simulink model "m5_das_ext"  (R2015b)
settings: Solver=FixedStepAuto  SolverMode=SingleTasking  StartTime=0.0  StopTime=10.0  RelTol=1e-3
undefined symbols (not defined in the file): DiscIntNeverNeededParam
libraries: simulink x5
settings Model: Creator=Capstone  LastModifiedBy=muscari.s

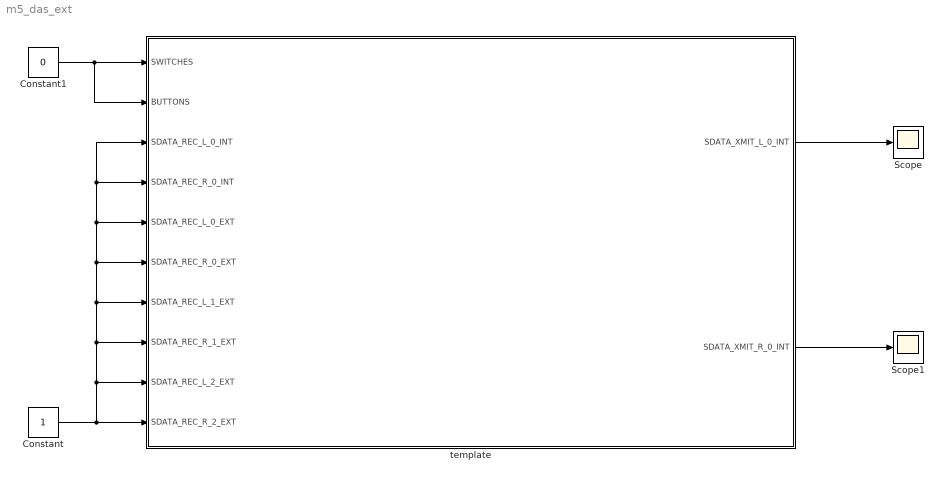
== system m5_das_ext ==
  Constant : Constant  OutDataTypeStr=int32  SampleTime=-1  LockScale=on
  Constant1 : Constant  Value=0  OutDataTypeStr=uint32  SampleTime=-1  LockScale=on
  Scope : Scope
  Scope1 : Scope
  template : Subsystem  TreatAsAtomicUnit=on
  wires:
  template/2(SDATA_XMIT_R_0_INT) -> Scope1/1
  template/1(SDATA_XMIT_L_0_INT) -> Scope/1
  Constant1/1 -> template/1(SWITCHES), template/2(BUTTONS)
  Constant/1 -> template/10(SDATA_REC_R_2_EXT), template/9(SDATA_REC_L_2_EXT), template/8(SDATA_REC_R_1_EXT), template/7(SDATA_REC_L_1_EXT), template/6(SDATA_REC_R_0_EXT), template/5(SDATA_REC_L_0_EXT), template/4(SDATA_REC_R_0_INT), template/3(SDATA_REC_L_0_INT)

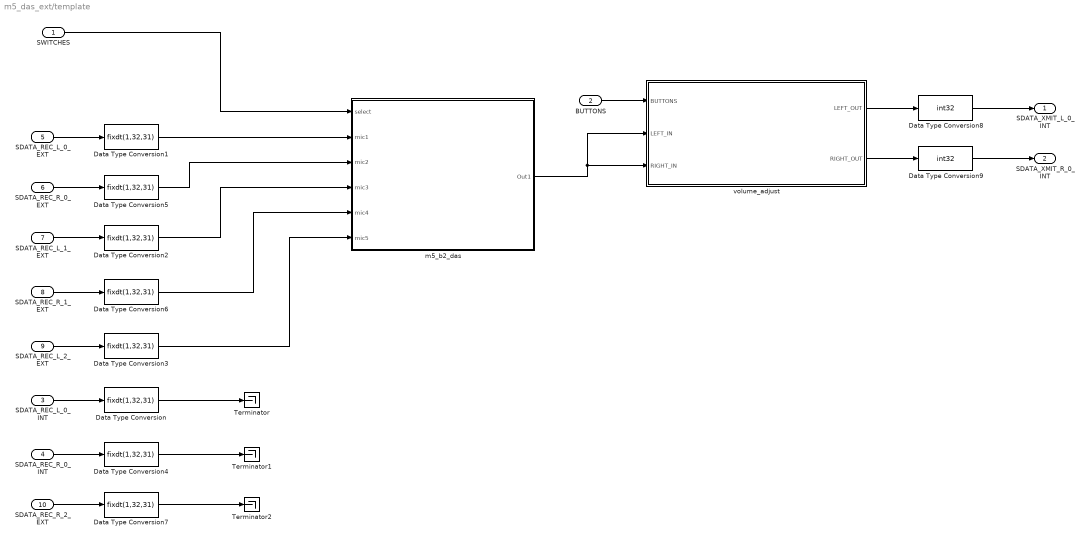
== system m5_das_ext/template ==
  SWITCHES : Inport
  BUTTONS : Inport  Port=2
  SDATA_REC_L_0_INT : Inport  Port=3
  SDATA_REC_R_0_INT : Inport  Port=4
  SDATA_REC_L_0_EXT : Inport  Port=5
  SDATA_REC_R_0_EXT : Inport  Port=6
  SDATA_REC_L_1_EXT : Inport  Port=7
  SDATA_REC_R_1_EXT : Inport  Port=8
  SDATA_REC_L_2_EXT : Inport  Port=9
  SDATA_REC_R_2_EXT : Inport  Port=10
  Data Type Conversion{,1..7} (8 alike) : DataTypeConversion  OutDataTypeStr=fixdt(1,32,31)  ConvertRealWorld=Stored Integer (SI)  RndMeth=Zero
  Data Type Conversion8 : DataTypeConversion  OutDataTypeStr=int32  ConvertRealWorld=Stored Integer (SI)  SaturateOnIntegerOverflow=on  RndMeth=Zero
  Data Type Conversion9 : DataTypeConversion  OutDataTypeStr=int32  ConvertRealWorld=Stored Integer (SI)  SaturateOnIntegerOverflow=on  RndMeth=Zero
  Terminator : Terminator
  Terminator1 : Terminator
  Terminator2 : Terminator
  m5_b2_das : Subsystem
  volume_adjust : Subsystem
  SDATA_XMIT_L_0_INT : Outport
  SDATA_XMIT_R_0_INT : Outport  Port=2
  wires:
  SDATA_REC_L_0_INT/1 -> Data Type Conversion/1
  SDATA_REC_R_0_INT/1 -> Data Type Conversion4/1
  SDATA_REC_L_0_EXT/1 -> Data Type Conversion1/1
  SDATA_REC_R_0_EXT/1 -> Data Type Conversion5/1
  SDATA_REC_L_1_EXT/1 -> Data Type Conversion2/1
  SDATA_REC_R_1_EXT/1 -> Data Type Conversion6/1
  SDATA_REC_L_2_EXT/1 -> Data Type Conversion3/1
  SDATA_REC_R_2_EXT/1 -> Data Type Conversion7/1
  BUTTONS/1 -> volume_adjust/1(BUTTONS)
  volume_adjust/1(LEFT_OUT) -> Data Type Conversion8/1
  volume_adjust/2(RIGHT_OUT) -> Data Type Conversion9/1
  Data Type Conversion8/1 -> SDATA_XMIT_L_0_INT/1
  Data Type Conversion9/1 -> SDATA_XMIT_R_0_INT/1
  SWITCHES/1 -> m5_b2_das/1(select)
  m5_b2_das/1(Out1) -> volume_adjust/2(LEFT_IN), volume_adjust/3(RIGHT_IN)
  Data Type Conversion7/1 -> Terminator2/1
  Data Type Conversion1/1 -> m5_b2_das/2(mic1)
  Data Type Conversion5/1 -> m5_b2_das/3(mic2)
  Data Type Conversion2/1 -> m5_b2_das/4(mic3)
  Data Type Conversion6/1 -> m5_b2_das/5(mic4)
  Data Type Conversion3/1 -> m5_b2_das/6(mic5)
  Data Type Conversion/1 -> Terminator/1
  Data Type Conversion4/1 -> Terminator1/1

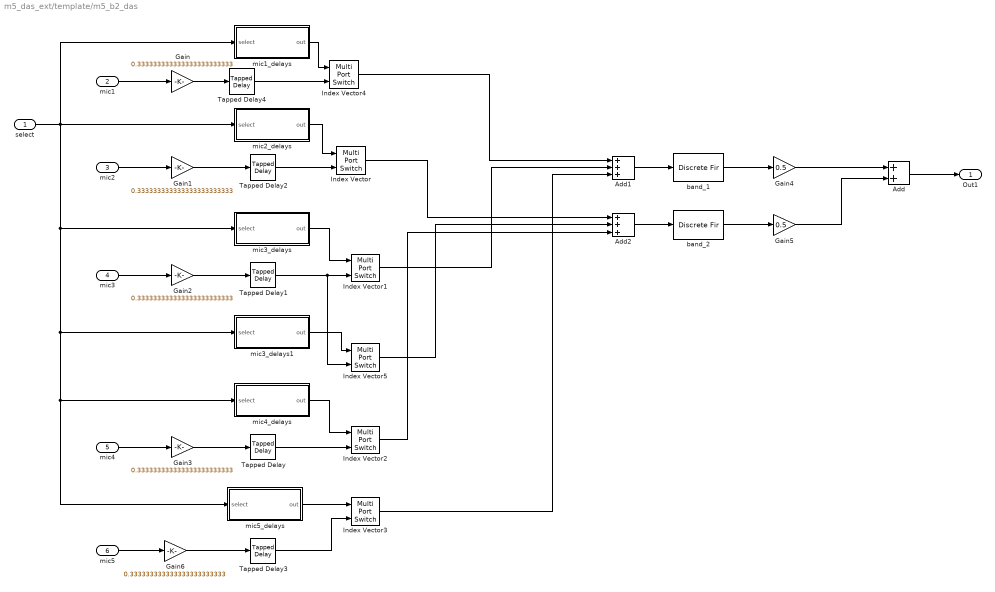
== system m5_das_ext/template/m5_b2_das ==
  select : Inport
  mic1 : Inport  Port=2
  mic2 : Inport  Port=3
  mic3 : Inport  Port=4
  mic4 : Inport  Port=5
  mic5 : Inport  Port=6
  Add : Sum  OutDataTypeStr=Inherit: Inherit via back propagation  RndMeth=Zero
  Add1 : Sum  Inputs=+++  OutDataTypeStr=Inherit: Inherit via back propagation  RndMeth=Zero
  Add2 : Sum  Inputs=+++  OutDataTypeStr=Inherit: Inherit via back propagation  RndMeth=Zero
  Gain{,1..3,6} (5 alike) : Gain  Gain=0.333333333333333333333333  ParamDataTypeStr=fixdt(1,32,31)  OutDataTypeStr=Inherit: Inherit via back propagation  RndMeth=Zero
  Gain4 : Gain  Gain=0.5  ParamDataTypeStr=fixdt(1,32,31)  OutDataTypeStr=Inherit: Inherit via back propagation  RndMeth=Zero
  Gain5 : Gain  Gain=0.5  ParamDataTypeStr=fixdt(1,32,31)  OutDataTypeStr=Inherit: Inherit via back propagation  RndMeth=Zero
  Index Vector{,1..5} (6 alike) : MultiPortSwitch  DataPortOrder=Zero-based contiguous  Inputs=1  zeroidx=on  OutDataTypeStr=Inherit: Inherit via back propagation  RndMeth=Zero
  Tapped Delay : simulink/Discrete/Tapped Delay  vinit=0.0  samptime=-1  NumDelays=17  DelayOrder=Newest  includeCurrent=on
  Tapped Delay1 : simulink/Discrete/Tapped Delay  vinit=0.0  samptime=-1  NumDelays=23  DelayOrder=Newest  includeCurrent=on
  Tapped Delay2 : simulink/Discrete/Tapped Delay  vinit=0.0  samptime=-1  NumDelays=17  DelayOrder=Newest  includeCurrent=on
  Tapped Delay3 : simulink/Discrete/Tapped Delay  vinit=0.0  samptime=-1  NumDelays=47  DelayOrder=Newest  includeCurrent=on
  Tapped Delay4 : simulink/Discrete/Tapped Delay  vinit=0.0  samptime=-1  NumDelays=47  DelayOrder=Newest  includeCurrent=on
  band_1 : DiscreteFir  FilterStructure=Direct form symmetric  Coefficients=[-0.0006782323736677226 -0.00061797501410385913 -0.00055397321805590496 -0.00048323247815375899 -0.0004028708790337593 -0.00031134760707579243 -0.00020971779606389519 -0.00010278232418469137 5.3436904881575911e-19 8.3960710390948516e-05 0.00012913286531009868 0.0001106975285270993 0 -0.00023387312629336585 -0.00062201085466718272 -0.0011931884772806989 -0.0019711128359718205 -0.0029715765047669592 -0.004199718624744401 -0.005647601071181548 -0.0072923056704523453 -0.0090947407353308349 -0.010999313649242089 -0.012934581980254817 -0.014814940943676075 -0.016543343055917401 -0.018014980247362096 -0.019121793633739462 -0.019757615819354583 -0.019823699110911527 -0.019234344027896737 -0.017922319003094409 -0.015843756286986907 -0.012982221866819705 -0.0093516886044415284 -0.004998190536744853 3.2646934950337606e-18 0.0055337554288432044 0.011466036402723352 0.017636310418650814 0.023866277092597258 0.029966655648355277 0.035744726086331557 0.041012267278278738 0.045593505981502414 0.049332682487998818 0.052100852097979732 0.053801576321740811 0.054375211888126766 0.053801576321740811 0.052100852097979732 0.049332682487998818 0.045593505981502414 0.041012267278278738 0.035744726086331557 0.029966655648355277 0.023866277092597258 0.017636310418650814 0.011466036402723352 0.0055337554288432044 3.2646934950337606e-18 -0.004998190536744853 -0.0093516886044415284 -0.012982221866819705 -0.015843756286986907 -0.017922319003094409 -0.019234344027896737 -0.019823699110911527 -0.019757615819354583 -0.019121793633739462 -0.018014980247362096 -0.016543343055917401 -0.014814940943676075 -0.012934581980254817 -0.010999313649242089 -0.0090947407353308349 -0.0072923056704523453 -0.005647601071181548 -0.004199718624744401 -0.0029715765047669592 -0.0019711128359718205 -0.0011931884772806989 -0.00062201085466718272 -0.00023387312629336585 0 0.0001106975285270993 0.00012913286531009868 8.3960710390948516e-05 5.3436904881575911e-19 -0.00010278232418469137 -0.00020971779606389519 -0.00031134760707579243 -0.0004028708790337593 -0.00048323247815375899 -0.00055397321805590496 -0.00061797501410385913 -0.0006782323736677226]  TapSumDataTypeStr=fixdt(true,33,31)  CoefDataTypeStr=fixdt(true,32,31)  ProductDataTypeStr=fixdt(true,32,31)  AccumDataTypeStr=fixdt(true,32,31)  OutDataTypeStr=fixdt(true,32,31)  RndMeth=Zero
  band_2 : DiscreteFir  FilterStructure=Direct form symmetric  Coefficients=[0.00031148187044047459 -5.1095487798674356e-05 -0.00038181538543607328 -0.00062770468081234799 -0.00074248208966874556 -0.00070004998252385145 -0.00051178880868063385 -0.00024029641821307493 1.3497652502458736e-18 6.2855354767847132e-05 -0.00018821474507956884 -0.00082507757949582753 -0.0018036973576697544 -0.0029373522174964005 -0.0039121114215135214 -0.0043514130535061441 -0.0039203448488945537 -0.0024435921126518823 3.3068411990632952e-18 0.0030435832447575401 0.0060838439066612541 0.008418897314846626 0.0094448958102664009 0.0088589350919107673 0.0068038414189030769 0.0038972922777800981 0.0011143345940897462 -0.00046666289418714551 6.8520344440706088e-18 0.0027988407275439764 0.0074343909211899992 0.01260813889409973 0.016432926965007474 0.016863521806897715 0.01225654659999127 0.0019235994936369317 -0.013475782186410821 -0.031831181698260456 -0.049836435118945893 -0.063583988307230208 -0.0693890532919961 -0.064664003280160934 -0.048634089538675054 -0.022707689666544836 0.0096145175855820303 0.043302394792267433 0.072729178597249478 0.09277940187005515 0.099888435657650002 0.09277940187005515 0.072729178597249478 0.043302394792267433 0.0096145175855820303 -0.022707689666544836 -0.048634089538675054 -0.064664003280160934 -0.0693890532919961 -0.063583988307230208 -0.049836435118945893 -0.031831181698260456 -0.013475782186410821 0.0019235994936369317 0.01225654659999127 0.016863521806897715 0.016432926965007474 0.01260813889409973 0.0074343909211899992 0.0027988407275439764 6.8520344440706088e-18 -0.00046666289418714551 0.0011143345940897462 0.0038972922777800981 0.0068038414189030769 0.0088589350919107673 0.0094448958102664009 0.008418897314846626 0.0060838439066612541 0.0030435832447575401 3.3068411990632952e-18 -0.0024435921126518823 -0.0039203448488945537 -0.0043514130535061441 -0.0039121114215135214 -0.0029373522174964005 -0.0018036973576697544 -0.00082507757949582753 -0.00018821474507956884 6.2855354767847132e-05 1.3497652502458736e-18 -0.00024029641821307493 -0.00051178880868063385 -0.00070004998252385145 -0.00074248208966874556 -0.00062770468081234799 -0.00038181538543607328 -5.1095487798674356e-05 0.00031148187044047459]  TapSumDataTypeStr=fixdt(true,33,31)  CoefDataTypeStr=fixdt(true,32,31)  ProductDataTypeStr=fixdt(true,32,31)  AccumDataTypeStr=fixdt(true,32,31)  OutDataTypeStr=fixdt(true,32,31)  RndMeth=Zero
  mic1_delays : Subsystem
  mic2_delays : Subsystem
  mic3_delays : Subsystem
  mic3_delays1 : Subsystem
  mic4_delays : Subsystem
  mic5_delays : Subsystem
  Out1 : Outport
  wires:
  mic1/1 -> Gain/1
  mic2/1 -> Gain1/1
  mic3/1 -> Gain2/1
  mic4/1 -> Gain3/1
  Gain1/1 -> Tapped Delay2/1
  Gain2/1 -> Tapped Delay1/1
  Gain3/1 -> Tapped Delay/1
  Tapped Delay2/1 -> Index Vector/2
  select/1 -> mic2_delays/1(select), mic1_delays/1(select), mic3_delays/1(select), mic3_delays1/1(select), mic4_delays/1(select), mic5_delays/1(select)
  Tapped Delay1/1 -> Index Vector5/2, Index Vector1/2
  Tapped Delay/1 -> Index Vector2/2
  band_1/1 -> Gain4/1
  band_2/1 -> Gain5/1
  Gain4/1 -> Add/1
  Gain5/1 -> Add/2
  mic5/1 -> Gain6/1
  Tapped Delay3/1 -> Index Vector3/2
  Add/1 -> Out1/1
  Gain6/1 -> Tapped Delay3/1
  Add1/1 -> band_1/1
  Add2/1 -> band_2/1
  Tapped Delay4/1 -> Index Vector4/2
  Gain/1 -> Tapped Delay4/1
  mic1_delays/1(out) -> Index Vector4/1
  Index Vector4/1 -> Add1/1
  mic3_delays/1(out) -> Index Vector1/1
  Index Vector1/1 -> Add1/2
  mic5_delays/1(out) -> Index Vector3/1
  Index Vector3/1 -> Add1/3
  mic2_delays/1(out) -> Index Vector/1
  mic4_delays/1(out) -> Index Vector2/1
  mic3_delays1/1(out) -> Index Vector5/1
  Index Vector5/1 -> Add2/2
  Index Vector/1 -> Add2/1
  Index Vector2/1 -> Add2/3

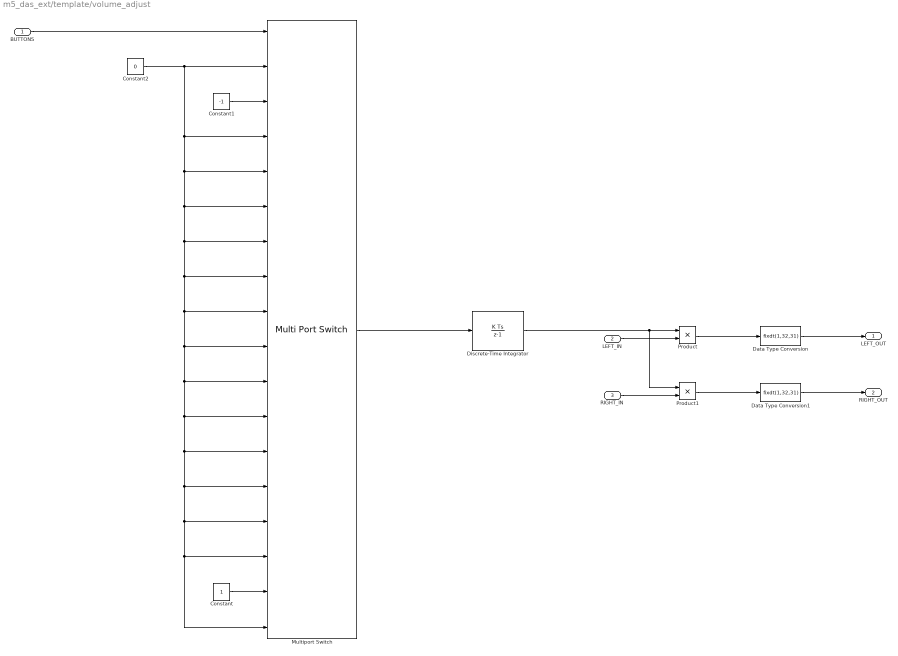
== system m5_das_ext/template/volume_adjust ==
  BUTTONS : Inport
  LEFT_IN : Inport  Port=2
  RIGHT_IN : Inport  Port=3
  Constant : Constant  OutDataTypeStr=fixdt(1,64,31)  SampleTime=-1
  Constant1 : Constant  Value=-1  OutDataTypeStr=fixdt(1,64,31)  SampleTime=-1
  Constant2 : Constant  Value=0  OutDataTypeStr=fixdt(1,64,31)  SampleTime=-1
  Data Type Conversion : DataTypeConversion  OutDataTypeStr=fixdt(1,32,31)  RndMeth=Zero
  Data Type Conversion1 : DataTypeConversion  OutDataTypeStr=fixdt(1,32,31)  RndMeth=Zero
  Discrete-Time Integrator : DiscreteIntegrator  gainval=0.00005  InitialCondition=1  OutDataTypeStr=fixdt(1,64,31)  RndMeth=Zero  SaturateOnIntegerOverflow=on  LimitOutput=on  UpperSaturationLimit=10000  LowerSaturationLimit=0  ICPrevOutput=DiscIntNeverNeededParam  ICPrevScaledInput=DiscIntNeverNeededParam
  Multiport Switch : MultiPortSwitch  Inputs=16  DataPortIndices={16,2}  DataPortForDefault=Additional data port  DiagnosticForDefault=None  OutDataTypeStr=Inherit: Inherit via back propagation  RndMeth=Zero
  Product : Product  OutDataTypeStr=Inherit: Inherit via back propagation  RndMeth=Zero
  Product1 : Product  OutDataTypeStr=Inherit: Inherit via back propagation  RndMeth=Zero
  LEFT_OUT : Outport
  RIGHT_OUT : Outport  Port=2
  wires:
  Multiport Switch/1 -> Discrete-Time Integrator/1
  BUTTONS/1 -> Multiport Switch/1
  Discrete-Time Integrator/1 -> Product1/1, Product/1
  LEFT_IN/1 -> Product/2
  RIGHT_IN/1 -> Product1/2
  Product/1 -> Data Type Conversion/1
  Product1/1 -> Data Type Conversion1/1
  Data Type Conversion/1 -> LEFT_OUT/1
  Data Type Conversion1/1 -> RIGHT_OUT/1
  Constant/1 -> Multiport Switch/17
  Constant1/1 -> Multiport Switch/3
  Constant2/1 -> Multiport Switch/2, Multiport Switch/18, Multiport Switch/16, Multiport Switch/15, Multiport Switch/14, Multiport Switch/13, Multiport Switch/12, Multiport Switch/11, Multiport Switch/10, Multiport Switch/9, Multiport Switch/8, Multiport Switch/7, Multiport Switch/6, Multiport Switch/5, Multiport Switch/4

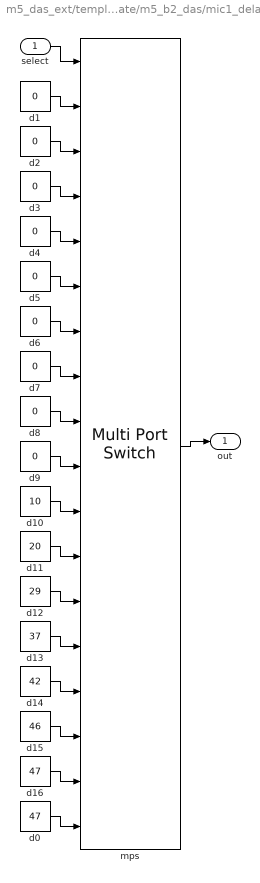
== system m5_das_ext/template/m5_b2_das/mic1_delays ==
  select : Inport
  d0 : Constant  Value=47  OutDataTypeStr=uint16  SampleTime=-1
  d{1..9} (9 alike) : Constant  Value=0  OutDataTypeStr=uint16  SampleTime=-1
  d10 : Constant  Value=10  OutDataTypeStr=uint16  SampleTime=-1
  d11 : Constant  Value=20  OutDataTypeStr=uint16  SampleTime=-1
  d12 : Constant  Value=29  OutDataTypeStr=uint16  SampleTime=-1
  d13 : Constant  Value=37  OutDataTypeStr=uint16  SampleTime=-1
  d14 : Constant  Value=42  OutDataTypeStr=uint16  SampleTime=-1
  d15 : Constant  Value=46  OutDataTypeStr=uint16  SampleTime=-1
  d16 : Constant  Value=47  OutDataTypeStr=uint16  SampleTime=-1
  mps : MultiPortSwitch  DataPortOrder=Zero-based contiguous  Inputs=16  DataPortForDefault=Additional data port  DiagnosticForDefault=None  OutDataTypeStr=Inherit: Inherit via back propagation  RndMeth=Zero  InputSameDT=on
  out : Outport
  wires:
  select/1 -> mps/1
  mps/1 -> out/1
  d1/1 -> mps/2
  d2/1 -> mps/3
  d3/1 -> mps/4
  d4/1 -> mps/5
  d5/1 -> mps/6
  d6/1 -> mps/7
  d7/1 -> mps/8
  d8/1 -> mps/9
  d9/1 -> mps/10
  d10/1 -> mps/11
  d11/1 -> mps/12
  d12/1 -> mps/13
  d13/1 -> mps/14
  d14/1 -> mps/15
  d15/1 -> mps/16
  d16/1 -> mps/17
  d0/1 -> mps/18

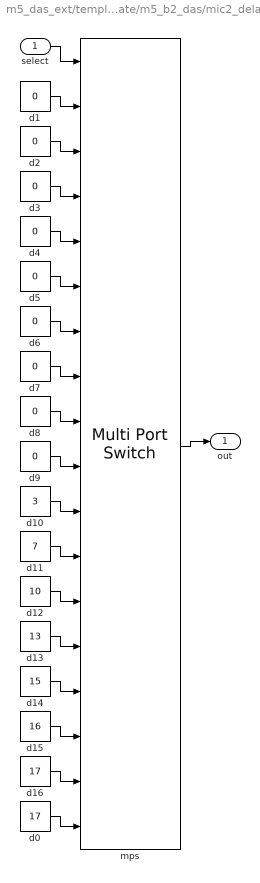
== system m5_das_ext/template/m5_b2_das/mic2_delays ==
  select : Inport
  d0 : Constant  Value=17  OutDataTypeStr=uint16  SampleTime=-1
  d{1..9} (9 alike) : Constant  Value=0  OutDataTypeStr=uint16  SampleTime=-1
  d10 : Constant  Value=3  OutDataTypeStr=uint16  SampleTime=-1
  d11 : Constant  Value=7  OutDataTypeStr=uint16  SampleTime=-1
  d12 : Constant  Value=10  OutDataTypeStr=uint16  SampleTime=-1
  d13 : Constant  Value=13  OutDataTypeStr=uint16  SampleTime=-1
  d14 : Constant  Value=15  OutDataTypeStr=uint16  SampleTime=-1
  d15 : Constant  Value=16  OutDataTypeStr=uint16  SampleTime=-1
  d16 : Constant  Value=17  OutDataTypeStr=uint16  SampleTime=-1
  mps : MultiPortSwitch  DataPortOrder=Zero-based contiguous  Inputs=16  DataPortForDefault=Additional data port  DiagnosticForDefault=None  OutDataTypeStr=Inherit: Inherit via back propagation  RndMeth=Zero  InputSameDT=on
  out : Outport
  wires:
  select/1 -> mps/1
  mps/1 -> out/1
  d1/1 -> mps/2
  d2/1 -> mps/3
  d3/1 -> mps/4
  d4/1 -> mps/5
  d5/1 -> mps/6
  d6/1 -> mps/7
  d7/1 -> mps/8
  d8/1 -> mps/9
  d9/1 -> mps/10
  d10/1 -> mps/11
  d11/1 -> mps/12
  d12/1 -> mps/13
  d13/1 -> mps/14
  d14/1 -> mps/15
  d15/1 -> mps/16
  d16/1 -> mps/17
  d0/1 -> mps/18

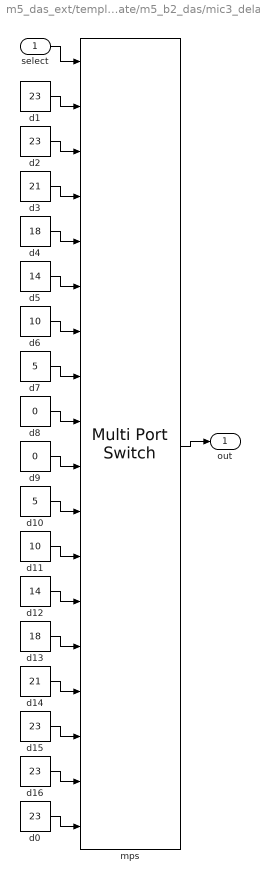
== system m5_das_ext/template/m5_b2_das/mic3_delays ==
  select : Inport
  d{0..2,15..16} (5 alike) : Constant  Value=23  OutDataTypeStr=uint16  SampleTime=-1
  d10 : Constant  Value=5  OutDataTypeStr=uint16  SampleTime=-1
  d11 : Constant  Value=10  OutDataTypeStr=uint16  SampleTime=-1
  d12 : Constant  Value=14  OutDataTypeStr=uint16  SampleTime=-1
  d13 : Constant  Value=18  OutDataTypeStr=uint16  SampleTime=-1
  d14 : Constant  Value=21  OutDataTypeStr=uint16  SampleTime=-1
  d3 : Constant  Value=21  OutDataTypeStr=uint16  SampleTime=-1
  d4 : Constant  Value=18  OutDataTypeStr=uint16  SampleTime=-1
  d5 : Constant  Value=14  OutDataTypeStr=uint16  SampleTime=-1
  d6 : Constant  Value=10  OutDataTypeStr=uint16  SampleTime=-1
  d7 : Constant  Value=5  OutDataTypeStr=uint16  SampleTime=-1
  d8 : Constant  Value=0  OutDataTypeStr=uint16  SampleTime=-1
  d9 : Constant  Value=0  OutDataTypeStr=uint16  SampleTime=-1
  mps : MultiPortSwitch  DataPortOrder=Zero-based contiguous  Inputs=16  DataPortForDefault=Additional data port  DiagnosticForDefault=None  OutDataTypeStr=Inherit: Inherit via back propagation  RndMeth=Zero  InputSameDT=on
  out : Outport
  wires:
  select/1 -> mps/1
  mps/1 -> out/1
  d1/1 -> mps/2
  d2/1 -> mps/3
  d3/1 -> mps/4
  d4/1 -> mps/5
  d5/1 -> mps/6
  d6/1 -> mps/7
  d7/1 -> mps/8
  d8/1 -> mps/9
  d9/1 -> mps/10
  d10/1 -> mps/11
  d11/1 -> mps/12
  d12/1 -> mps/13
  d13/1 -> mps/14
  d14/1 -> mps/15
  d15/1 -> mps/16
  d16/1 -> mps/17
  d0/1 -> mps/18

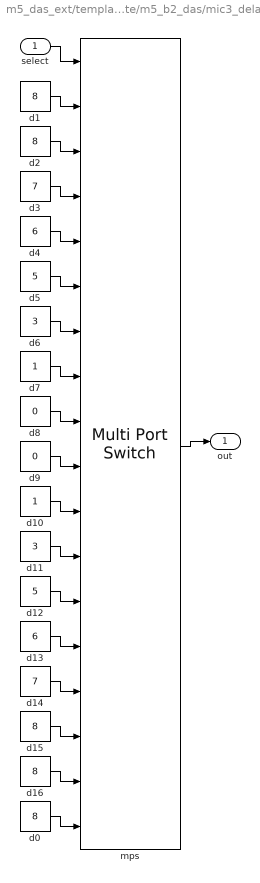
== system m5_das_ext/template/m5_b2_das/mic3_delays1 ==
  select : Inport
  d{0..2,15..16} (5 alike) : Constant  Value=8  OutDataTypeStr=uint16  SampleTime=-1
  d10 : Constant  OutDataTypeStr=uint16  SampleTime=-1
  d11 : Constant  Value=3  OutDataTypeStr=uint16  SampleTime=-1
  d12 : Constant  Value=5  OutDataTypeStr=uint16  SampleTime=-1
  d13 : Constant  Value=6  OutDataTypeStr=uint16  SampleTime=-1
  d14 : Constant  Value=7  OutDataTypeStr=uint16  SampleTime=-1
  d3 : Constant  Value=7  OutDataTypeStr=uint16  SampleTime=-1
  d4 : Constant  Value=6  OutDataTypeStr=uint16  SampleTime=-1
  d5 : Constant  Value=5  OutDataTypeStr=uint16  SampleTime=-1
  d6 : Constant  Value=3  OutDataTypeStr=uint16  SampleTime=-1
  d7 : Constant  OutDataTypeStr=uint16  SampleTime=-1
  d8 : Constant  Value=0  OutDataTypeStr=uint16  SampleTime=-1
  d9 : Constant  Value=0  OutDataTypeStr=uint16  SampleTime=-1
  mps : MultiPortSwitch  DataPortOrder=Zero-based contiguous  Inputs=16  DataPortForDefault=Additional data port  DiagnosticForDefault=None  OutDataTypeStr=Inherit: Inherit via back propagation  RndMeth=Zero  InputSameDT=on
  out : Outport
  wires:
  select/1 -> mps/1
  mps/1 -> out/1
  d1/1 -> mps/2
  d2/1 -> mps/3
  d3/1 -> mps/4
  d4/1 -> mps/5
  d5/1 -> mps/6
  d6/1 -> mps/7
  d7/1 -> mps/8
  d8/1 -> mps/9
  d9/1 -> mps/10
  d10/1 -> mps/11
  d11/1 -> mps/12
  d12/1 -> mps/13
  d13/1 -> mps/14
  d14/1 -> mps/15
  d15/1 -> mps/16
  d16/1 -> mps/17
  d0/1 -> mps/18

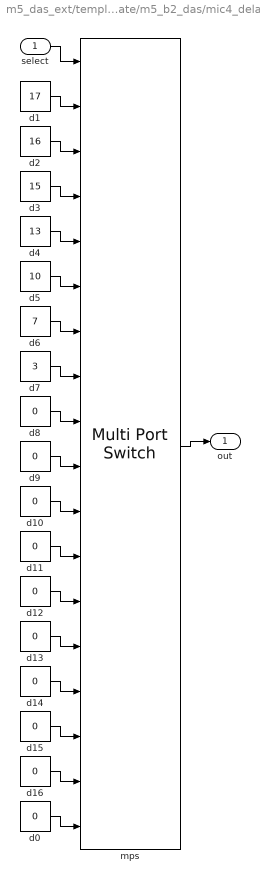
== system m5_das_ext/template/m5_b2_das/mic4_delays ==
  select : Inport
  d{0,8..16} (10 alike) : Constant  Value=0  OutDataTypeStr=uint16  SampleTime=-1
  d1 : Constant  Value=17  OutDataTypeStr=uint16  SampleTime=-1
  d2 : Constant  Value=16  OutDataTypeStr=uint16  SampleTime=-1
  d3 : Constant  Value=15  OutDataTypeStr=uint16  SampleTime=-1
  d4 : Constant  Value=13  OutDataTypeStr=uint16  SampleTime=-1
  d5 : Constant  Value=10  OutDataTypeStr=uint16  SampleTime=-1
  d6 : Constant  Value=7  OutDataTypeStr=uint16  SampleTime=-1
  d7 : Constant  Value=3  OutDataTypeStr=uint16  SampleTime=-1
  mps : MultiPortSwitch  DataPortOrder=Zero-based contiguous  Inputs=16  DataPortForDefault=Additional data port  DiagnosticForDefault=None  OutDataTypeStr=Inherit: Inherit via back propagation  RndMeth=Zero  InputSameDT=on
  out : Outport
  wires:
  select/1 -> mps/1
  mps/1 -> out/1
  d1/1 -> mps/2
  d2/1 -> mps/3
  d3/1 -> mps/4
  d4/1 -> mps/5
  d5/1 -> mps/6
  d6/1 -> mps/7
  d7/1 -> mps/8
  d8/1 -> mps/9
  d9/1 -> mps/10
  d10/1 -> mps/11
  d11/1 -> mps/12
  d12/1 -> mps/13
  d13/1 -> mps/14
  d14/1 -> mps/15
  d15/1 -> mps/16
  d16/1 -> mps/17
  d0/1 -> mps/18

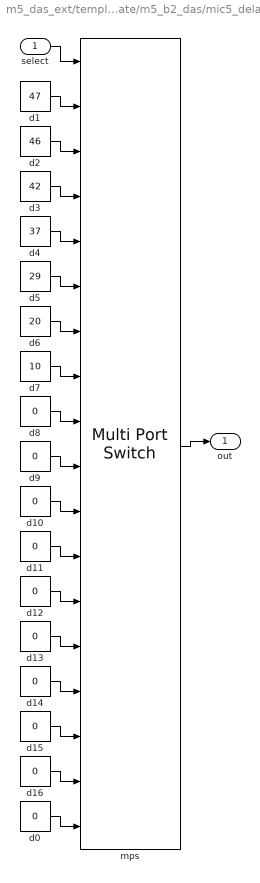
== system m5_das_ext/template/m5_b2_das/mic5_delays ==
  select : Inport
  d{0,8..16} (10 alike) : Constant  Value=0  OutDataTypeStr=uint16  SampleTime=-1
  d1 : Constant  Value=47  OutDataTypeStr=uint16  SampleTime=-1
  d2 : Constant  Value=46  OutDataTypeStr=uint16  SampleTime=-1
  d3 : Constant  Value=42  OutDataTypeStr=uint16  SampleTime=-1
  d4 : Constant  Value=37  OutDataTypeStr=uint16  SampleTime=-1
  d5 : Constant  Value=29  OutDataTypeStr=uint16  SampleTime=-1
  d6 : Constant  Value=20  OutDataTypeStr=uint16  SampleTime=-1
  d7 : Constant  Value=10  OutDataTypeStr=uint16  SampleTime=-1
  mps : MultiPortSwitch  DataPortOrder=Zero-based contiguous  Inputs=16  DataPortForDefault=Additional data port  DiagnosticForDefault=None  OutDataTypeStr=Inherit: Inherit via back propagation  RndMeth=Zero  InputSameDT=on
  out : Outport
  wires:
  select/1 -> mps/1
  mps/1 -> out/1
  d1/1 -> mps/2
  d2/1 -> mps/3
  d3/1 -> mps/4
  d4/1 -> mps/5
  d5/1 -> mps/6
  d6/1 -> mps/7
  d7/1 -> mps/8
  d8/1 -> mps/9
  d9/1 -> mps/10
  d10/1 -> mps/11
  d11/1 -> mps/12
  d12/1 -> mps/13
  d13/1 -> mps/14
  d14/1 -> mps/15
  d15/1 -> mps/16
  d16/1 -> mps/17
  d0/1 -> mps/18
